simulink model "LAB_04_17_OCT_SIM_KIN"  (R2022b)
settings: Solver=ode3  StartTime=0.0  StopTime=100  FixedStep=0.1  RelTol=1e-3
values from neighbouring files (symbols this model uses):
  A0 = diag([1 1 1])    [LAB_04_17_OCT_MAT_KIN.m]    (also in LAB_05_24_OCT_MAT_KIN_COSDIR.m; LAB_06.m = A_target_fun(0); core_attitude_test.m = eye(3,3); lab_07_MAT.m)
  I = [Ix 0 0 ... (first row only)    [LAB_03_3_OCT_MAT_EUL_2_VERIFICATION.m]    (also in LAB_03_3_OCT_MAT_EUL_DOUBLESPIN.m = diag([Ix, Iy, Iz]); LAB_03_3_OCT_MAT_EUL_SPINAXIS.m = diag([Ix, Iy, Iz]); LAB_03_3_OCT_MAT_EUL_VECT.m; LAB_04_17_OCT_MAT_KIN.m)
  om_0 = [om_x0, om_y0, om_z0]    [LAB_03_3_OCT_MAT_EUL.m]    (also in LAB_03_3_OCT_MAT_EUL_2_VERIFICATION.m = [om_x0; om_y0; om_z0]; LAB_03_3_OCT_MAT_EUL_DOUBLESPIN.m = [om_x0; om_y0; om_z0]; LAB_03_3_OCT_MAT_EUL_SPINAXIS.m = [om_x0; om_y0; om_z0]; LAB_03_3_OCT_MAT_EUL_VECT.m = [om_x0; om_y0; om_z0])
libraries: sharedutil x1, matrix_library x1
settings Model: Creator=maria  LastModifiedBy=maria

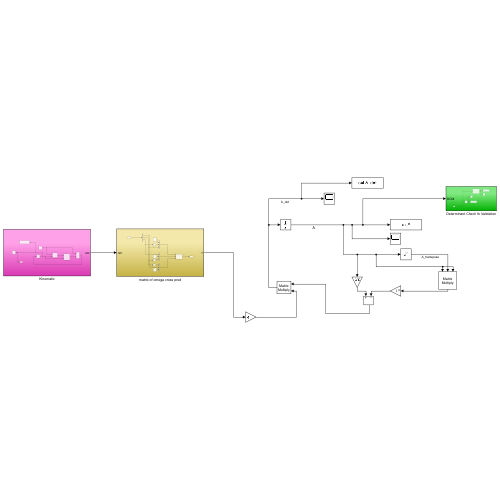
[thumbnail: Simulink's stored preview of the top-level diagram]
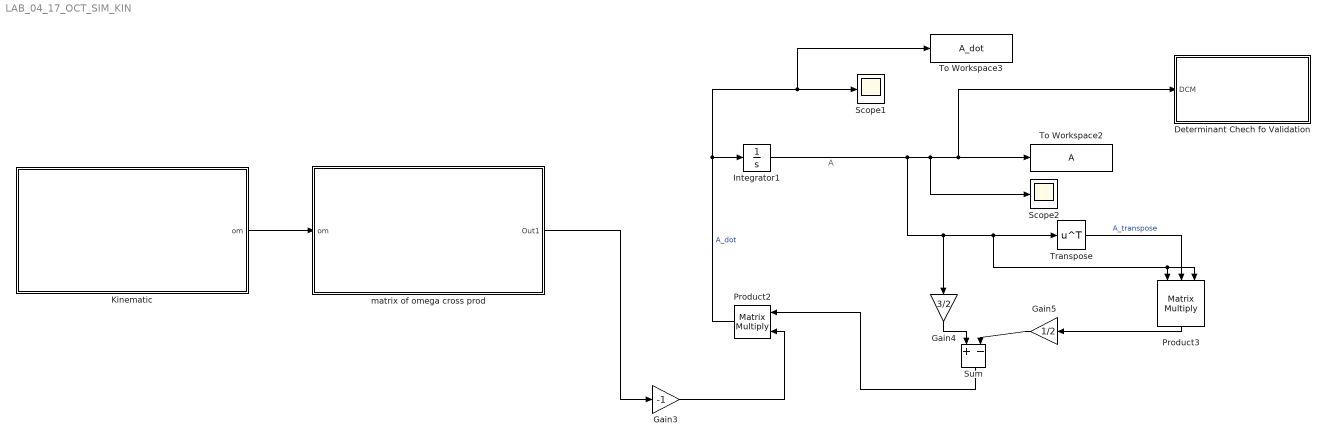
== system LAB_04_17_OCT_SIM_KIN ==
  note: A
  Determinant Chech fo Validation : Subsystem
  Gain3 : Gain  Gain=-1
  Gain4 : Gain  Gain=3/2
  Gain5 : Gain  Gain=1/2
  Integrator1 : Integrator  InitialCondition=A0
  Kinematic : Subsystem
  Product2 : Product  Multiplication=Matrix(*)
  Product3 : Product  Inputs=3  Multiplication=Matrix(*)
  Scope1 : Scope
  Scope2 : Scope
  Sum : Sum  Inputs=+-
  To Workspace2 : ToWorkspace  VariableName=A  SampleTime=-1
  To Workspace3 : ToWorkspace  VariableName=A_dot  SampleTime=-1
  Transpose : Math  Operator=transpose
  matrix of omega cross prod : Subsystem
  wires:
  Integrator1/1 -> Gain4/1, Product3/3, Product3/1, Transpose/1, Scope2/1, Determinant Chech fo Validation/1(DCM), To Workspace2/1
  Gain3/1 -> Product2/2
  Product2/1 -> Integrator1/1, To Workspace3/1, Scope1/1  "A_dot"
  Transpose/1 -> Product3/2  "A_transpose"
  Gain4/1 -> Sum/1
  Gain5/1 -> Sum/2
  Product3/1 -> Gain5/1
  Sum/1 -> Product2/1
  matrix of omega cross prod/1(Out1) -> Gain3/1
  Kinematic/1(om) -> matrix of omega cross prod/1(om)

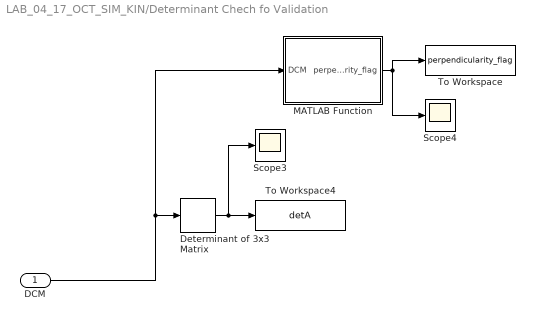
== system LAB_04_17_OCT_SIM_KIN/Determinant Chech fo Validation ==
  DCM : Inport
  Determinant of 3x3 Matrix : sharedutil/Determinant of 3x3 Matrix  aMode=aMode
      settings: LibrarySourceBlock=|
      | aerolibutil/Determinant of
      | 3x3 Matrix
  MATLAB Function : MATLAB Function  TreatAsAtomicUnit=on
  Scope3 : Scope
  Scope4 : Scope
  To Workspace : ToWorkspace  VariableName=perpendicularity_flag  SampleTime=-1
  To Workspace4 : ToWorkspace  VariableName=detA  SampleTime=-1
  wires:
  Determinant of 3x3 Matrix/1 -> Scope3/1, To Workspace4/1
  DCM/1 -> MATLAB Function/1(DCM), Determinant of 3x3 Matrix/1
  MATLAB Function/1(perpendicularity_flag) -> To Workspace/1, Scope4/1

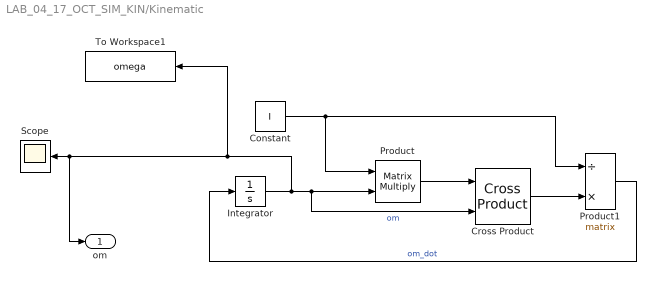
== system LAB_04_17_OCT_SIM_KIN/Kinematic ==
  Constant : Constant  Value=I
  Cross Product : matrix_library/Cross Product
  Integrator : Integrator  InitialCondition=om_0
  Product : Product  Multiplication=Matrix(*)
  Product1 : Product  Inputs=/*  Multiplication=Matrix(*)
  Scope : Scope
  To Workspace1 : ToWorkspace  VariableName=omega  SampleTime=-1
  om : Outport
  wires:
  Constant/1 -> Product/1, Product1/1
  Integrator/1 -> To Workspace1/1, om/1, Scope/1, Product/2, Cross Product/2  "om"
  Product1/1 -> Integrator/1  "om_dot"
  Product/1 -> Cross Product/1
  Cross Product/1 -> Product1/2

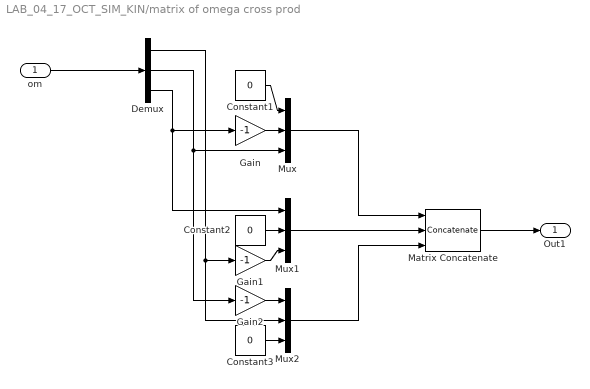
== system LAB_04_17_OCT_SIM_KIN/matrix of omega cross prod ==
  om : Inport
  Constant1 : Constant  Value=0
  Constant2 : Constant  Value=0
  Constant3 : Constant  Value=0
  Demux : Demux  Outputs=3
  Gain : Gain  Gain=-1
  Gain1 : Gain  Gain=-1
  Gain2 : Gain  Gain=-1
  Matrix Concatenate : Concatenate  NumInputs=3  Mode=Multidimensional array  ConcatenateDimension=2
  Mux : Mux  Inputs=3
  Mux1 : Mux  Inputs=3
  Mux2 : Mux  Inputs=3
  Out1 : Outport
  wires:
  Matrix Concatenate/1 -> Out1/1
  Demux/1 -> Gain1/1, Mux2/2
  Mux1/1 -> Matrix Concatenate/2
  Constant3/1 -> Mux2/3
  Gain/1 -> Mux/2
  Gain2/1 -> Mux2/1
  Constant1/1 -> Mux/1
  Demux/3 -> Gain/1, Mux1/1
  Demux/2 -> Mux/3, Gain2/1
  Mux/1 -> Matrix Concatenate/1
  Gain1/1 -> Mux1/3
  Mux2/1 -> Matrix Concatenate/3
  Constant2/1 -> Mux1/2
  om/1 -> Demux/1

== matlab function LAB_04_17_OCT_SIM_KIN/Determinant Chech fo Validation/MATLAB Function ==
  data: DCM input; perpendicularity_flag output
function perpendicularity_flag = fcn(DCM)


perpendicularity_flag =zeros(3,1);

    x   = DCM(1,:);
    y   = DCM(2,:);
    z   = DCM(3,:);

    perpendicularity_flag(1)=dot(x,y);
    perpendicularity_flag(2)=dot(x,z);
    perpendicularity_flag(1)=dot(z,y);

end
